simulink library "casper_library_downconverter"  (Simulink 7.0)
libraries: xbsIndex_r4 x81, casper_library_downconverter x18, casper_library_misc x1
(part 1 of 2)
settings Model: Creator=mdexter  LastModifiedBy=mdexter

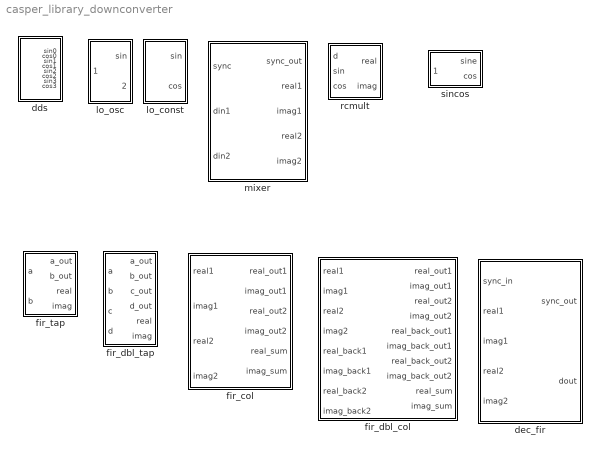
== system casper_library_downconverter ==
  dds : Subsystem  mask(dds){freq_div=4, freq=1, num_lo=4, n_bits=8, latency=2}
      mask prompts: freq_div "Frequency divisions (M)"; freq "Frequency (? / M*2pi)"; num_lo "Parallel LOs"; n_bits "Bit Width"
      mask help:
      | Generates P channels of sin and cos data for mixing
      | with input data in a DDC. To generate frequency
      | N/M(Fc x P) (where Fc is the clock rate)
      | M = "Frequency Divisions", N = "Frequency",
      | Parallel LOs = P
      mask init:
      | dds_init(gcb, ...
      |     'freq_div', freq_div, ...
      |     'freq', freq, ...
      |     'num_lo', num_lo, ...
      |     'n_bits', n_bits, ...
      |     'latency', latency);
      settings: AttributesFormatString=lo at -1/4
      mask Help: eval('xlWeb(''http://casper.berkeley.edu/wiki/Dds'')')
  dec_fir : Subsystem  mask(dec_fir){n_inputs=2, coeff=getfield( getfield( get_param( gcb,'UserData' ), 'parameters'),'coeff'), n_bits=4, quantization=Truncate, add_latency=1, mult_latency=2, coeff_bit_width=25, coeff_bin_pt=24, adder_tree_hdl=on}
      mask prompts: n_inputs "Number of Parallel Streams"; coeff "Coefficients"; n_bits "Bit Width Out"; quantization "Quantization Behavior"; add_latency "Add Latency"; mult_latency "Mult Latency"; coeff_bit_width "Coefficient bit width"; coeff_bin_pt "Coefficient binary point"; adder_tree_hdl "Implement first stage of adder trees after multiplication as behavioural HDL"
      mask help: FIR filter which can handle multiple time samples in parallel and decimates down to 1 time sample. If coefficients are symmetric, will automatically fold before multiplying.
      mask init:
      | dec_fir_init(gcb, ...
      |     'n_inputs', n_inputs, ...
      |     'coeff', coeff, ...
      |     'n_bits', n_bits, ...
      |     'quantization', quantization, ...
      |     'add_latency', add_latency, ...
      |     'mult_latency', mult_latency, ...
      |     'coeff_bit_width', coeff_bit_width, ...
      |     'coeff_bin_pt', coeff_bin_pt, ...
      |     'adder_tree_hdl', adder_tree_hdl);
      settings: AttributesFormatString=|
      | 8 taps
      | 4_3 r/i
      mask Help: eval('xlWeb(''http://casper.berkeley.edu/wiki/Dec_fir'')')
      mask StyleString: edit,edit,edit,popup(Truncate|Round  (unbiased: +/- Inf)|Round  (unbiased: Even Values)),edit,edit,edit,edit,checkbox
  fir_col : Subsystem  mask(fir_col){n_inputs=2, coeff=[2 3], add_latency=1, mult_latency=2, coeff_bit_width=25, coeff_bin_pt=24, adder_tree_hdl=off}
      mask prompts: n_inputs "Inputs"; coeff "Coefficients"; add_latency "Add latency"; mult_latency "Mult Latency"; coeff_bit_width "Coefficient bit width"; coeff_bin_pt "Coefficient binary point"; adder_tree_hdl "Implement first stage of adder trees on output as behavioural HDL"
      mask init:
      | fir_col_init(gcb, ...
      |     'n_inputs', n_inputs,...
      |     'coeff', coeff, ...
      |     'mult_latency', mult_latency, ...
      |     'add_latency', add_latency, ...
      |     'coeff_bit_width', coeff_bit_width, ...
      |     'coeff_bin_pt', coeff_bin_pt, ...
      |     'adder_tree_hdl', adder_tree_hdl);
      mask Help: eval('xlWeb(''http://casper.berkeley.edu/wiki/Fir_col'')')
  fir_dbl_col : Subsystem  mask(fir_dbl_col){n_inputs=2, coeff=[0.1 0.2 0.3 0.4], add_latency=1, mult_latency=2, coeff_bit_width=25, coeff_bin_pt=24, adder_tree_hdl=off}
      mask prompts: n_inputs "Inputs"; coeff "Coefficients"; add_latency "Add latency"; mult_latency "Mult Latency"; coeff_bit_width "Coefficient bit width"; coeff_bin_pt "Coefficient binary point"; adder_tree_hdl "Implement first stage of adder trees on output as behavioural HDL"
      mask init:
      | fir_dbl_col_init(gcb, ...
      |     'n_inputs', n_inputs, ...
      |     'coeff', coeff, ...
      |     'mult_latency', mult_latency, ...
      |     'add_latency', add_latency, ...
      |     'coeff_bit_width', coeff_bit_width, ...
      |     'coeff_bin_pt', coeff_bin_pt,  ...
      |     'adder_tree_hdl', adder_tree_hdl);
      mask Help: eval('xlWeb(''http://casper.berkeley.edu/wiki/Fir_dbl_col'')')
  fir_dbl_tap : Subsystem  mask(fir_dbl_tap){factor=0.073384, add_latency=1, mult_latency=2, coeff_bit_width=18, coeff_bin_pt=17}
      mask prompts: add_latency "Add latency"; mult_latency "Mult latency"; coeff_bit_width "Coefficient bit width"; coeff_bin_pt "Coefficient binary point"
      mask Help: eval('xlWeb(''http://casper.berkeley.edu/wiki/Fir_dbl_tap'')')
  fir_tap : Subsystem  mask(fir_tap){factor=1, latency=2, coeff_bit_width=25, coeff_bin_pt=24}
      mask prompts: latency "Mult latency"; coeff_bit_width "Coefficient bit width"; coeff_bin_pt "Coefficient binary point"
      mask help: Multiplies input data with factor specified.
      mask Help: eval('xlWeb(''http://casper.berkeley.edu/wiki/Fir_tap'')')
  lo_const : Subsystem  mask(lo_const){n_bits=18, phase=0}
      mask prompts: n_bits "Output Bitwidth"; phase "Phase (0 to 2*pi)"
      mask help:
      | Generates a complex constant associated with the
      | phase supplied as a parameter.
      mask Help: eval('xlWeb(''http://casper.berkeley.edu/wiki/Lo_const'')')
  lo_osc : Subsystem  mask(lo_osc){n_bits=7, counter_step=3, counter_start=4, counter_width=4, latency=2}
      mask prompts: n_bits "Output Bitwidth"; counter_step "counter step"; counter_start "counter start value"; counter_width "Counter Bitwidth"; latency "Lookup latency"
      mask help:
      | Generates -sin and cos data using a look-up
      | table.
      mask init:
      | lo_osc_init(gcb, ...
      |     'n_bits', n_bits, ...
      |     'counter_step', counter_step, ...
      |     'counter_start', counter_start, ...
      |     'counter_width', counter_width, ...
      |     'latency', latency);
      mask Help: eval('xlWeb(''http://casper.berkeley.edu/wiki/Lo_osc'')')
  mixer : Subsystem  mask(mixer){freq_div=2, freq=2, nstreams=2, n_bits=4, bram_latency=2, mult_latency=4}
      mask prompts: freq_div "Frequency Divisions (M)"; freq "Mixing Frequency (? / M*2pi)"; nstreams "Number of Parallel Streams"; n_bits "Bit Width"; bram_latency "BRAM Latency"; mult_latency "Mult Latency"
      mask help: Digitally mixes an input signal (which can be several samples in parallel) with an LO of the indicated frequency (which is some fraction of the native FPGA clock rate).
      mask init:
      | mixer_init(gcb, ...
      |     'freq_div', freq_div, ...
      |     'freq', freq, ...
      |     'nstreams', nstreams, ...
      |     'n_bits', n_bits, ...
      |     'bram_latency', bram_latency, ...
      |     'mult_latency', mult_latency);
      settings: AttributesFormatString=lo at -2/2
      mask Help: eval('xlWeb(''http://casper.berkeley.edu/wiki/Mixer'')')
  rcmult : Subsystem  mask(rcmult){latency=3}
      mask prompts: latency "Multiplier latency"
      mask help:
      | Multiplies input data with cos and sin inputs and
      | outputs results on real and imag ports
      | respectively.
      mask Help: eval('xlWeb(''http://casper.berkeley.edu/wiki/Rcmult'')')
  sincos : Subsystem  mask(sincos){func=sine and cosine, neg_sin=off, neg_cos=off, symmetric=on, handle_sync=off, depth_bits=10, bit_width=16, bram_latency=2}
      mask prompts: func "Function"; neg_sin "Negative sine"; neg_cos "Negative cosine"; symmetric "Symmetric output"; handle_sync "Handle sync"; depth_bits "Lookup table depth (2^?)"; bit_width "Output bit width"; bram_latency "BRAM latency"
      mask init:
      | sincos_init(gcb, ...
      |     'func', func, ...
      |     'neg_sin', neg_sin, ...
      |     'neg_cos', neg_cos, ...
      |     'symmetric', symmetric, ...
      |     'handle_sync', handle_sync, ...
      |     'depth_bits', depth_bits, ...
      |     'bit_width', bit_width, ...
      |     'bram_latency', bram_latency);
      mask StyleString: popup(cosine|sine|sine and cosine),checkbox,checkbox,checkbox,checkbox,edit,edit,edit

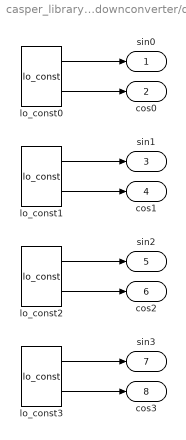
== system casper_library_downconverter/dds ==
  lo_const0 : casper_library_downconverter/lo_const  SystemSampleTime=-1  n_bits=8  phase=0
  lo_const1 : casper_library_downconverter/lo_const  SystemSampleTime=-1  n_bits=8  phase=1.5708
  lo_const2 : casper_library_downconverter/lo_const  SystemSampleTime=-1  n_bits=8  phase=3.1416
  lo_const3 : casper_library_downconverter/lo_const  SystemSampleTime=-1  n_bits=8  phase=4.7124
  sin0 : Outport  OutDataType=sfix(16)  OutScaling=2^0
  cos0 : Outport  Port=2  OutDataType=sfix(16)  OutScaling=2^0
  sin1 : Outport  Port=3  OutDataType=sfix(16)  OutScaling=2^0
  cos1 : Outport  Port=4  OutDataType=sfix(16)  OutScaling=2^0
  sin2 : Outport  Port=5  OutDataType=sfix(16)  OutScaling=2^0
  cos2 : Outport  Port=6  OutDataType=sfix(16)  OutScaling=2^0
  sin3 : Outport  Port=7  OutDataType=sfix(16)  OutScaling=2^0
  cos3 : Outport  Port=8  OutDataType=sfix(16)  OutScaling=2^0
  wires:
  lo_const3/2 -> cos3/1
  lo_const3/1 -> sin3/1
  lo_const2/2 -> cos2/1
  lo_const2/1 -> sin2/1
  lo_const1/2 -> cos1/1
  lo_const1/1 -> sin1/1
  lo_const0/2 -> cos0/1
  lo_const0/1 -> sin0/1

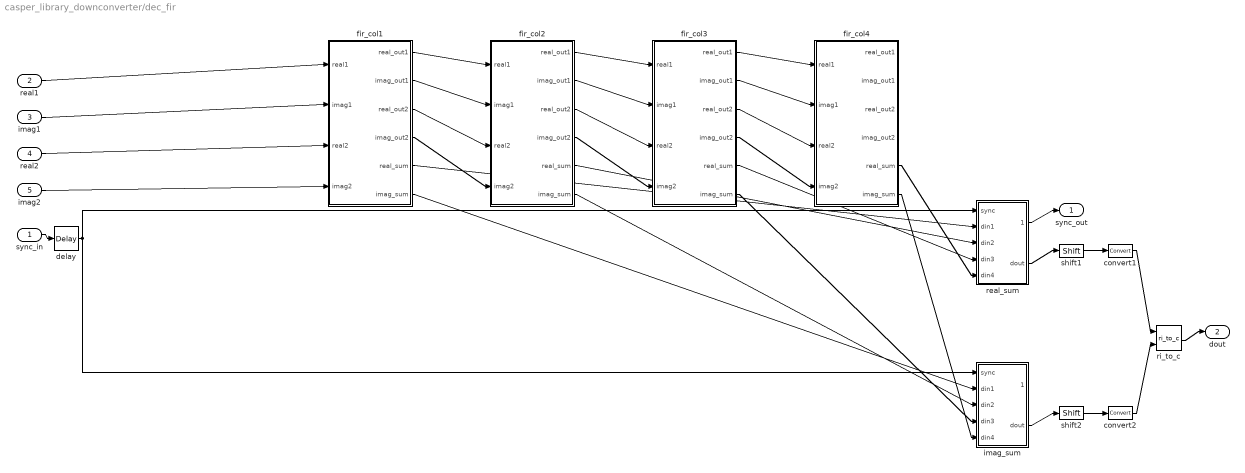
== system casper_library_downconverter/dec_fir ==
  sync_in : Inport
  real1 : Inport  Port=2
  imag1 : Inport  Port=3
  real2 : Inport  Port=4
  imag2 : Inport  Port=5
  convert1 : xbsIndex_r4/Convert  arith_type="Signed  (2's comp)"  n_bits=4  bin_pt=3  quantization=Truncate  overflow=Wrap  latency=1  dbl_ovrd=off  pipeline=off  block_type=convert
      settings: block_version=10.1.3
  convert2 : xbsIndex_r4/Convert  arith_type="Signed  (2's comp)"  n_bits=4  bin_pt=3  quantization=Truncate  overflow=Wrap  latency=1  dbl_ovrd=off  pipeline=off  block_type=convert
      settings: block_version=10.1.3
  delay : xbsIndex_r4/Delay  en=off  latency=4  dbl_ovrd=off  reg_retiming=off  block_type=delay
  fir_col1 : Subsystem  AncestorBlock=casper_library_downconverter/fir_col  mask(fir_col){n_inputs=2, coeff=[0.20000000000000001110223024625157     0.10000000000000000555111512312578], add_latency=1, mult_latency=2, coeff_bit_width=25, coeff_bin_pt=24, adder_tree_hdl=on}
      mask prompts: n_inputs "Inputs"; coeff "Coefficients"; add_latency "Add latency"; mult_latency "Mult Latency"; coeff_bit_width "Coefficient bit width"; coeff_bin_pt "Coefficient binary point"; adder_tree_hdl "Implement first stage of adder trees on output as behavioural HDL"
      mask init: same as casper_library_downconverter/fir_col
      mask Help: eval('xlWeb(''http://casper.berkeley.edu/wiki/Fir_col'')')
  fir_col2 : Subsystem  AncestorBlock=casper_library_downconverter/fir_col  mask(fir_col){n_inputs=2, coeff=[0.40000000000000002220446049250313     0.29999999999999998889776975374843], add_latency=1, mult_latency=2, coeff_bit_width=25, coeff_bin_pt=24, adder_tree_hdl=on}
      mask prompts: n_inputs "Inputs"; coeff "Coefficients"; add_latency "Add latency"; mult_latency "Mult Latency"; coeff_bit_width "Coefficient bit width"; coeff_bin_pt "Coefficient binary point"; adder_tree_hdl "Implement first stage of adder trees on output as behavioural HDL"
      mask init: same as casper_library_downconverter/fir_col
      mask Help: eval('xlWeb(''http://casper.berkeley.edu/wiki/Fir_col'')')
  fir_col3 : Subsystem  AncestorBlock=casper_library_downconverter/fir_col  mask(fir_col){n_inputs=2, coeff=[0.59999999999999997779553950749687                                    0.5], add_latency=1, mult_latency=2, coeff_bit_width=25, coeff_bin_pt=24, adder_tree_hdl=on}
      mask prompts: n_inputs "Inputs"; coeff "Coefficients"; add_latency "Add latency"; mult_latency "Mult Latency"; coeff_bit_width "Coefficient bit width"; coeff_bin_pt "Coefficient binary point"; adder_tree_hdl "Implement first stage of adder trees on output as behavioural HDL"
      mask init: same as casper_library_downconverter/fir_col
      mask Help: eval('xlWeb(''http://casper.berkeley.edu/wiki/Fir_col'')')
  fir_col4 : Subsystem  AncestorBlock=casper_library_downconverter/fir_col  mask(fir_col){n_inputs=2, coeff=[0.80000000000000004440892098500626     0.69999999999999995559107901499374], add_latency=1, mult_latency=2, coeff_bit_width=25, coeff_bin_pt=24, adder_tree_hdl=on}
      mask prompts: n_inputs "Inputs"; coeff "Coefficients"; add_latency "Add latency"; mult_latency "Mult Latency"; coeff_bit_width "Coefficient bit width"; coeff_bin_pt "Coefficient binary point"; adder_tree_hdl "Implement first stage of adder trees on output as behavioural HDL"
      mask init: same as casper_library_downconverter/fir_col
      mask Help: eval('xlWeb(''http://casper.berkeley.edu/wiki/Fir_col'')')
  imag_sum : Subsystem  AncestorBlock=casper_library_misc/adder_tree  mask(adder_tree){n_inputs=4, latency=1, first_stage_hdl=off, behavioral=off}
      mask prompts: n_inputs "Number of Inputs"; latency "Add Latency"; first_stage_hdl "Use behavioural HDL for first stage of adders"; behavioral "Use behavioral HDL for all adders"
      mask help:
      | Sums all inputs using a tree of adds and delays.
      |
      | Number of inputs: The number of inputs to the block to be summed
      | Add latency: The number of clock cycles to perform one addition (affects timing).
      | Use behavioural HDL for first stage of adders: Causes the first stage of adders to be absorbed into DSP blocks if multipliers precede them (Virtex 5).
      | Use behavioural HDL for all adders: Causes all adders in all stages to be implemented in behavioural HDL (may improve timing).
      mask init:
      | adder_tree_init(gcb, ...
      |     'n_inputs', n_inputs, ...
      |     'latency', latency, ...
      |     'first_stage_hdl', first_stage_hdl, ...
      |     'behavioral', behavioral);
      settings: AttributesFormatString=latency 2
      mask Help: eval('xlWeb(''http://casper.berkeley.edu/wiki/Adder_tree'')')
  real_sum : Subsystem  AncestorBlock=casper_library_misc/adder_tree  mask(adder_tree){n_inputs=4, latency=1, first_stage_hdl=off, behavioral=off}
      mask prompts: n_inputs "Number of Inputs"; latency "Add Latency"; first_stage_hdl "Use behavioural HDL for first stage of adders"; behavioral "Use behavioral HDL for all adders"
      mask help:
      | Sums all inputs using a tree of adds and delays.
      |
      | Number of inputs: The number of inputs to the block to be summed
      | Add latency: The number of clock cycles to perform one addition (affects timing).
      | Use behavioural HDL for first stage of adders: Causes the first stage of adders to be absorbed into DSP blocks if multipliers precede them (Virtex 5).
      | Use behavioural HDL for all adders: Causes all adders in all stages to be implemented in behavioural HDL (may improve timing).
      mask init:
      | adder_tree_init(gcb, ...
      |     'n_inputs', n_inputs, ...
      |     'latency', latency, ...
      |     'first_stage_hdl', first_stage_hdl, ...
      |     'behavioral', behavioral);
      settings: AttributesFormatString=latency 2
      mask Help: eval('xlWeb(''http://casper.berkeley.edu/wiki/Adder_tree'')')
  ri_to_c : casper_library_misc/ri_to_c  SystemSampleTime=-1
  shift1 : xbsIndex_r4/Shift  shift_dir=Left  shift_bits=1  en=off  latency=0  precision=Full  arith_type="Signed  (2's comp)"  n_bits=16  bin_pt=14  quantization=Truncate  overflow=Wrap  dbl_ovrd=off  block_type=shift
      settings: block_version=10.1.3
  shift2 : xbsIndex_r4/Shift  shift_dir=Left  shift_bits=1  en=off  latency=0  precision=Full  arith_type="Signed  (2's comp)"  n_bits=16  bin_pt=14  quantization=Truncate  overflow=Wrap  dbl_ovrd=off  block_type=shift
      settings: block_version=10.1.3
  sync_out : Outport
  dout : Outport  Port=2
  wires:
  real_sum/1(sync_out) -> sync_out/1
  delay/1 -> imag_sum/1(sync), real_sum/1(sync)
  sync_in/1 -> delay/1
  ri_to_c/1 -> dout/1
  convert2/1 -> ri_to_c/2
  convert1/1 -> ri_to_c/1
  shift2/1 -> convert2/1
  shift1/1 -> convert1/1
  imag_sum/2(dout) -> shift2/1
  real_sum/2(dout) -> shift1/1
  fir_col4/6(imag_sum) -> imag_sum/5(din4)
  fir_col4/5(real_sum) -> real_sum/5(din4)
  fir_col3/4(imag_out2) -> fir_col4/4(imag2)
  fir_col3/3(real_out2) -> fir_col4/3(real2)
  fir_col3/2(imag_out1) -> fir_col4/2(imag1)
  fir_col3/1(real_out1) -> fir_col4/1(real1)
  fir_col3/6(imag_sum) -> imag_sum/4(din3)
  fir_col3/5(real_sum) -> real_sum/4(din3)
  fir_col2/4(imag_out2) -> fir_col3/4(imag2)
  fir_col2/3(real_out2) -> fir_col3/3(real2)
  fir_col2/2(imag_out1) -> fir_col3/2(imag1)
  fir_col2/1(real_out1) -> fir_col3/1(real1)
  fir_col2/6(imag_sum) -> imag_sum/3(din2)
  fir_col2/5(real_sum) -> real_sum/3(din2)
  fir_col1/4(imag_out2) -> fir_col2/4(imag2)
  fir_col1/3(real_out2) -> fir_col2/3(real2)
  fir_col1/2(imag_out1) -> fir_col2/2(imag1)
  fir_col1/1(real_out1) -> fir_col2/1(real1)
  fir_col1/6(imag_sum) -> imag_sum/2(din1)
  fir_col1/5(real_sum) -> real_sum/2(din1)
  imag2/1 -> fir_col1/4(imag2)
  real2/1 -> fir_col1/3(real2)
  imag1/1 -> fir_col1/2(imag1)
  real1/1 -> fir_col1/1(real1)

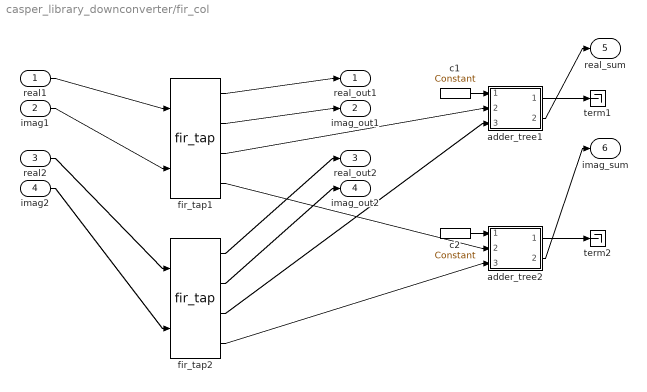
== system casper_library_downconverter/fir_col ==
  real1 : Inport
  imag1 : Inport  Port=2
  real2 : Inport  Port=3
  imag2 : Inport  Port=4
  adder_tree1 : Subsystem  AncestorBlock=casper_library_misc/adder_tree  mask(adder_tree){n_inputs=2, latency=1, first_stage_hdl=off, behavioral=off}
      mask prompts: n_inputs "Number of Inputs"; latency "Add Latency"; first_stage_hdl "Use behavioural HDL for first stage of adders"; behavioral "Use behavioral HDL for all adders"
      mask help:
      | Sums all inputs using a tree of adds and delays.
      |
      | Number of inputs: The number of inputs to the block to be summed
      | Add latency: The number of clock cycles to perform one addition (affects timing).
      | Use behavioural HDL for first stage of adders: Causes the first stage of adders to be absorbed into DSP blocks if multipliers precede them (Virtex 5).
      | Use behavioural HDL for all adders: Causes all adders in all stages to be implemented in behavioural HDL (may improve timing).
      mask init:
      | adder_tree_init(gcb, ...
      |     'n_inputs', n_inputs, ...
      |     'latency', latency, ...
      |     'first_stage_hdl', first_stage_hdl, ...
      |     'behavioral', behavioral);
      settings: AttributesFormatString=latency 1
      mask Help: eval('xlWeb(''http://casper.berkeley.edu/wiki/Adder_tree'')')
  adder_tree2 : Subsystem  AncestorBlock=casper_library_misc/adder_tree  mask(adder_tree){n_inputs=2, latency=1, first_stage_hdl=off, behavioral=off}
      mask prompts: n_inputs "Number of Inputs"; latency "Add Latency"; first_stage_hdl "Use behavioural HDL for first stage of adders"; behavioral "Use behavioral HDL for all adders"
      mask help:
      | Sums all inputs using a tree of adds and delays.
      |
      | Number of inputs: The number of inputs to the block to be summed
      | Add latency: The number of clock cycles to perform one addition (affects timing).
      | Use behavioural HDL for first stage of adders: Causes the first stage of adders to be absorbed into DSP blocks if multipliers precede them (Virtex 5).
      | Use behavioural HDL for all adders: Causes all adders in all stages to be implemented in behavioural HDL (may improve timing).
      mask init:
      | adder_tree_init(gcb, ...
      |     'n_inputs', n_inputs, ...
      |     'latency', latency, ...
      |     'first_stage_hdl', first_stage_hdl, ...
      |     'behavioral', behavioral);
      settings: AttributesFormatString=latency 1
      mask Help: eval('xlWeb(''http://casper.berkeley.edu/wiki/Adder_tree'')')
  c1 : xbsIndex_r4/Constant  arith_type=Signed (2's comp)  const=1  n_bits=16  bin_pt=14  explicit_period=on  period=1  equ=P=C  opselect=C  inp2=PCIN>>17  opr=+  inp1=P  carry=CIN  dbl_ovrd=off  block_type=constant
  c2 : xbsIndex_r4/Constant  arith_type=Signed (2's comp)  const=1  n_bits=16  bin_pt=14  explicit_period=on  period=1  equ=P=C  opselect=C  inp2=PCIN>>17  opr=+  inp1=P  carry=CIN  dbl_ovrd=off  block_type=constant
  fir_tap1 : casper_library_downconverter/fir_tap  SystemSampleTime=-1  factor=2  latency=2  coeff_bit_width=25  coeff_bin_pt=24
  fir_tap2 : casper_library_downconverter/fir_tap  SystemSampleTime=-1  factor=3  latency=2  coeff_bit_width=25  coeff_bin_pt=24
  term1 : Terminator
  term2 : Terminator
  real_out1 : Outport
  imag_out1 : Outport  Port=2
  real_out2 : Outport  Port=3
  imag_out2 : Outport  Port=4
  real_sum : Outport  Port=5
  imag_sum : Outport  Port=6
  wires:
  adder_tree1/1(sync_out) -> term1/1
  adder_tree2/1(sync_out) -> term2/1
  c1/1 -> adder_tree1/1(sync)
  c2/1 -> adder_tree2/1(sync)
  adder_tree1/2(dout) -> real_sum/1
  adder_tree2/2(dout) -> imag_sum/1
  real1/1 -> fir_tap1/1
  imag1/1 -> fir_tap1/2
  fir_tap1/1 -> real_out1/1
  fir_tap1/2 -> imag_out1/1
  fir_tap1/3 -> adder_tree1/2(din1)
  fir_tap1/4 -> adder_tree2/2(din1)
  real2/1 -> fir_tap2/1
  imag2/1 -> fir_tap2/2
  fir_tap2/1 -> real_out2/1
  fir_tap2/2 -> imag_out2/1
  fir_tap2/3 -> adder_tree1/3(din2)
  fir_tap2/4 -> adder_tree2/3(din2)

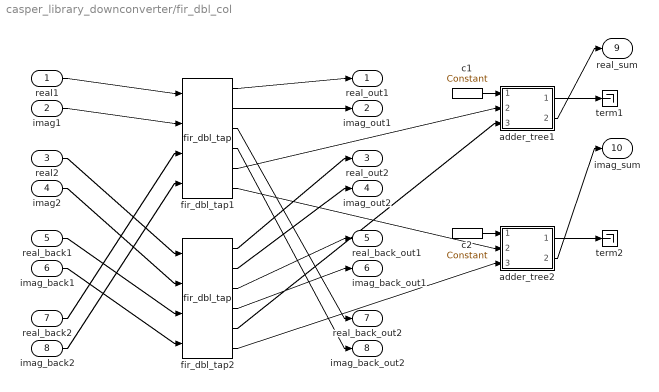
== system casper_library_downconverter/fir_dbl_col ==
  real1 : Inport
  imag1 : Inport  Port=2
  real2 : Inport  Port=3
  imag2 : Inport  Port=4
  real_back1 : Inport  Port=5
  imag_back1 : Inport  Port=6
  real_back2 : Inport  Port=7
  imag_back2 : Inport  Port=8
  adder_tree1 : Subsystem  AncestorBlock=casper_library_misc/adder_tree  mask(adder_tree){n_inputs=2, latency=1, first_stage_hdl=off, behavioral=off}
      mask prompts: n_inputs "Number of Inputs"; latency "Add Latency"; first_stage_hdl "Use behavioural HDL for first stage of adders"; behavioral "Use behavioral HDL for all adders"
      mask help:
      | Sums all inputs using a tree of adds and delays.
      |
      | Number of inputs: The number of inputs to the block to be summed
      | Add latency: The number of clock cycles to perform one addition (affects timing).
      | Use behavioural HDL for first stage of adders: Causes the first stage of adders to be absorbed into DSP blocks if multipliers precede them (Virtex 5).
      | Use behavioural HDL for all adders: Causes all adders in all stages to be implemented in behavioural HDL (may improve timing).
      mask init:
      | adder_tree_init(gcb, ...
      |     'n_inputs', n_inputs, ...
      |     'latency', latency, ...
      |     'first_stage_hdl', first_stage_hdl, ...
      |     'behavioral', behavioral);
      settings: AttributesFormatString=latency 1
      mask Help: eval('xlWeb(''http://casper.berkeley.edu/wiki/Adder_tree'')')
  adder_tree2 : Subsystem  AncestorBlock=casper_library_misc/adder_tree  mask(adder_tree){n_inputs=2, latency=1, first_stage_hdl=off, behavioral=off}
      mask prompts: n_inputs "Number of Inputs"; latency "Add Latency"; first_stage_hdl "Use behavioural HDL for first stage of adders"; behavioral "Use behavioral HDL for all adders"
      mask help:
      | Sums all inputs using a tree of adds and delays.
      |
      | Number of inputs: The number of inputs to the block to be summed
      | Add latency: The number of clock cycles to perform one addition (affects timing).
      | Use behavioural HDL for first stage of adders: Causes the first stage of adders to be absorbed into DSP blocks if multipliers precede them (Virtex 5).
      | Use behavioural HDL for all adders: Causes all adders in all stages to be implemented in behavioural HDL (may improve timing).
      mask init:
      | adder_tree_init(gcb, ...
      |     'n_inputs', n_inputs, ...
      |     'latency', latency, ...
      |     'first_stage_hdl', first_stage_hdl, ...
      |     'behavioral', behavioral);
      settings: AttributesFormatString=latency 1
      mask Help: eval('xlWeb(''http://casper.berkeley.edu/wiki/Adder_tree'')')
  c1 : xbsIndex_r4/Constant  arith_type=Signed (2's comp)  const=1  n_bits=16  bin_pt=14  explicit_period=on  period=1  equ=P=C  opselect=C  inp2=PCIN>>17  opr=+  inp1=P  carry=CIN  dbl_ovrd=off  block_type=constant
  c2 : xbsIndex_r4/Constant  arith_type=Signed (2's comp)  const=1  n_bits=16  bin_pt=14  explicit_period=on  period=1  equ=P=C  opselect=C  inp2=PCIN>>17  opr=+  inp1=P  carry=CIN  dbl_ovrd=off  block_type=constant
  fir_dbl_tap1 : casper_library_downconverter/fir_dbl_tap  SystemSampleTime=-1  factor=0.1  add_latency=1  mult_latency=2  coeff_bit_width=25  coeff_bin_pt=24
  fir_dbl_tap2 : casper_library_downconverter/fir_dbl_tap  SystemSampleTime=-1  factor=0.2  add_latency=1  mult_latency=2  coeff_bit_width=25  coeff_bin_pt=24
  term1 : Terminator
  term2 : Terminator
  real_out1 : Outport
  imag_out1 : Outport  Port=2
  real_out2 : Outport  Port=3
  imag_out2 : Outport  Port=4
  real_back_out1 : Outport  Port=5
  imag_back_out1 : Outport  Port=6
  real_back_out2 : Outport  Port=7
  imag_back_out2 : Outport  Port=8
  real_sum : Outport  Port=9
  imag_sum : Outport  Port=10
  wires:
  adder_tree1/1(sync_out) -> term1/1
  adder_tree2/1(sync_out) -> term2/1
  c1/1 -> adder_tree1/1(sync)
  c2/1 -> adder_tree2/1(sync)
  adder_tree1/2(dout) -> real_sum/1
  adder_tree2/2(dout) -> imag_sum/1
  real1/1 -> fir_dbl_tap1/1
  imag1/1 -> fir_dbl_tap1/2
  real_back2/1 -> fir_dbl_tap1/3
  imag_back2/1 -> fir_dbl_tap1/4
  fir_dbl_tap1/1 -> real_out1/1
  fir_dbl_tap1/2 -> imag_out1/1
  fir_dbl_tap1/3 -> real_back_out2/1
  fir_dbl_tap1/4 -> imag_back_out2/1
  fir_dbl_tap1/5 -> adder_tree1/2(din1)
  fir_dbl_tap1/6 -> adder_tree2/2(din1)
  real2/1 -> fir_dbl_tap2/1
  imag2/1 -> fir_dbl_tap2/2
  real_back1/1 -> fir_dbl_tap2/3
  imag_back1/1 -> fir_dbl_tap2/4
  fir_dbl_tap2/1 -> real_out2/1
  fir_dbl_tap2/2 -> imag_out2/1
  fir_dbl_tap2/3 -> real_back_out1/1
  fir_dbl_tap2/4 -> imag_back_out1/1
  fir_dbl_tap2/5 -> adder_tree1/3(din2)
  fir_dbl_tap2/6 -> adder_tree2/3(din2)

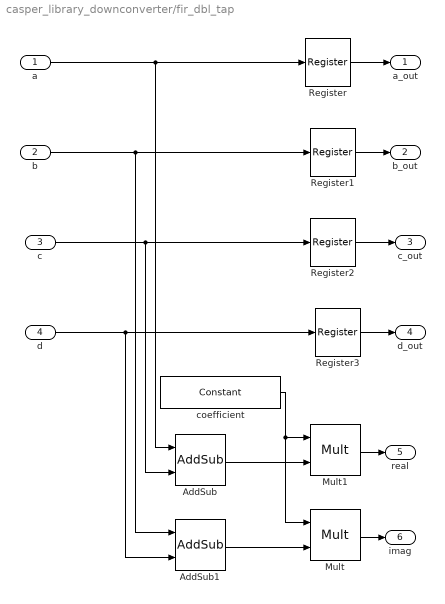
== system casper_library_downconverter/fir_dbl_tap ==
  a : Inport  OutDataType=sfix(16)  OutScaling=2^0
  b : Inport  Port=2  OutDataType=sfix(16)  OutScaling=2^0
  c : Inport  Port=3  OutDataType=sfix(16)  OutScaling=2^0
  d : Inport  Port=4  OutDataType=sfix(16)  OutScaling=2^0
  AddSub : xbsIndex_r4/AddSub  mode=Addition  use_carryin=off  use_carryout=off  en=off  latency=add_latency  precision=Full  arith_type="Signed  (2's comp)"  n_bits=18  bin_pt=16  quantization=Truncate  overflow=Wrap  dbl_ovrd=off  use_behavioral_HDL=on  pipelined=off  use_rpm=on  hw_selection=Fabric  block_type=addsub
      settings: xl_area=[0, 0, 0, 0, 0, 0, 0]  block_version=9.2.01
  AddSub1 : xbsIndex_r4/AddSub  mode=Addition  use_carryin=off  use_carryout=off  en=off  latency=add_latency  precision=Full  arith_type="Signed  (2's comp)"  n_bits=18  bin_pt=16  quantization=Truncate  overflow=Wrap  dbl_ovrd=off  use_behavioral_HDL=on  pipelined=off  use_rpm=on  hw_selection=Fabric  block_type=addsub
      settings: xl_area=[0, 0, 0, 0, 0, 0, 0]  block_version=9.2.01
  Mult : xbsIndex_r4/Mult  precision=Full  arith_type="Signed  (2's comp)"  n_bits=18  bin_pt=17  quantization=Truncate  overflow=Wrap  en=off  latency=mult_latency  dbl_ovrd=off  use_behavioral_HDL=on  use_embedded=on  opt=Speed  optimum_pipeline=off  pipeline=on  use_rpm=off  placement_style=Rectangular shape  block_type=mult
      settings: infoedit=Hardware notes: To use the internal pipeline stage of the dedicated multiplier you must select 'Pipeline for maximum performance'.  xl_area=[0, 0, 0, 0, 0, 0, 0]  block_version=9.2.01
  Mult1 : xbsIndex_r4/Mult  precision=Full  arith_type="Signed  (2's comp)"  n_bits=18  bin_pt=17  quantization=Truncate  overflow=Wrap  en=off  latency=mult_latency  dbl_ovrd=off  use_behavioral_HDL=on  use_embedded=on  opt=Speed  optimum_pipeline=off  pipeline=on  use_rpm=off  placement_style=Rectangular shape  block_type=mult
      settings: infoedit=Hardware notes: To use the internal pipeline stage of the dedicated multiplier you must select 'Pipeline for maximum performance'.  xl_area=[0, 0, 0, 0, 0, 0, 0]  block_version=9.2.01
  Register{,1..3} (4 alike) : xbsIndex_r4/Register  init=0  rst=off  en=off  dbl_ovrd=off  block_type=register
      settings: xl_area=[0, 0, 0, 0, 0, 0, 0]  block_version=9.2.01
  coefficient : xbsIndex_r4/Constant  arith_type=Signed (2's comp)  const=factor  n_bits=coeff_bit_width  bin_pt=coeff_bin_pt  explicit_period=on  period=1  equ=P=C  opselect=C  inp2=PCIN>>17  opr=+  inp1=P  carry=CIN  dbl_ovrd=off  block_type=constant
      settings: block_version=9.2.01
  a_out : Outport  OutDataType=sfix(16)  OutScaling=2^0
  b_out : Outport  Port=2  OutDataType=sfix(16)  OutScaling=2^0
  c_out : Outport  Port=3  OutDataType=sfix(16)  OutScaling=2^0
  d_out : Outport  Port=4  OutDataType=sfix(16)  OutScaling=2^0
  real : Outport  Port=5  OutDataType=sfix(16)  OutScaling=2^0
  imag : Outport  Port=6  OutDataType=sfix(16)  OutScaling=2^0
  wires:
  AddSub1/1 -> Mult/2
  AddSub/1 -> Mult1/2
  d/1 -> AddSub1/2, Register3/1
  c/1 -> AddSub/2, Register2/1
  b/1 -> AddSub1/1, Register1/1
  a/1 -> AddSub/1, Register/1
  Register2/1 -> c_out/1
  Register3/1 -> d_out/1
  Mult1/1 -> real/1
  Mult/1 -> imag/1
  coefficient/1 -> Mult1/1, Mult/1
  Register/1 -> a_out/1
  Register1/1 -> b_out/1

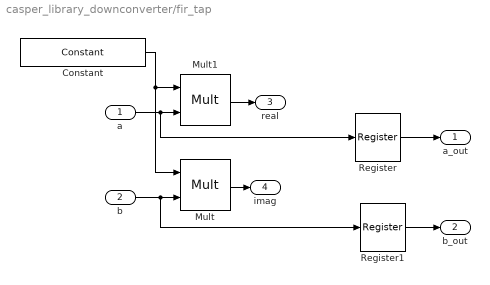
== system casper_library_downconverter/fir_tap ==
  a : Inport  OutDataType=sfix(16)  OutScaling=2^0
  b : Inport  Port=2  OutDataType=sfix(16)  OutScaling=2^0
  Constant : xbsIndex_r4/Constant  arith_type=Signed (2's comp)  const=factor  n_bits=coeff_bit_width  bin_pt=coeff_bin_pt  explicit_period=on  period=1  equ=P=C  opselect=C  inp2=PCIN>>17  opr=+  inp1=P  carry=CIN  dbl_ovrd=off  block_type=constant
      settings: block_version=9.1.01
  Mult : xbsIndex_r4/Mult  precision=Full  arith_type="Signed  (2's comp)"  n_bits=18  bin_pt=17  quantization=Truncate  overflow=Wrap  en=off  latency=latency  dbl_ovrd=off  use_behavioral_HDL=on  use_embedded=on  opt=Speed  optimum_pipeline=off  pipeline=on  use_rpm=off  placement_style=Rectangular shape  block_type=mult
      settings: infoedit=Hardware notes: To use the internal pipeline stage of the dedicated multiplier you must select 'Pipeline for maximum performance'.  xl_area=[0, 0, 0, 0, 0, 0, 0]  block_version=9.1.01
  Mult1 : xbsIndex_r4/Mult  precision=Full  arith_type="Signed  (2's comp)"  n_bits=18  bin_pt=17  quantization=Truncate  overflow=Wrap  en=off  latency=latency  dbl_ovrd=off  use_behavioral_HDL=on  use_embedded=on  opt=Speed  optimum_pipeline=off  pipeline=on  use_rpm=off  placement_style=Rectangular shape  block_type=mult
      settings: infoedit=Hardware notes: To use the internal pipeline stage of the dedicated multiplier you must select 'Pipeline for maximum performance'.  xl_area=[0, 0, 0, 0, 0, 0, 0]  block_version=9.1.01
  Register : xbsIndex_r4/Register  init=0  rst=off  en=off  dbl_ovrd=off  block_type=register
      settings: xl_area=[0, 0, 0, 0, 0, 0, 0]  block_version=9.1.01
  Register1 : xbsIndex_r4/Register  init=0  rst=off  en=off  dbl_ovrd=off  block_type=register
      settings: xl_area=[0, 0, 0, 0, 0, 0, 0]  block_version=9.1.01
  a_out : Outport  OutDataType=sfix(16)  OutScaling=2^0
  b_out : Outport  Port=2  OutDataType=sfix(16)  OutScaling=2^0
  real : Outport  Port=3  OutDataType=sfix(16)  OutScaling=2^0
  imag : Outport  Port=4  OutDataType=sfix(16)  OutScaling=2^0
  wires:
  Mult1/1 -> real/1
  b/1 -> Mult/2, Register1/1
  Mult/1 -> imag/1
  a/1 -> Mult1/2, Register/1
  Constant/1 -> Mult1/1, Mult/1
  Register/1 -> a_out/1
  Register1/1 -> b_out/1

== system casper_library_downconverter/lo_const ==
  const : xbsIndex_r4/Constant  arith_type=Signed (2's comp)  const=real(exp(phase*1j))  n_bits=n_bits  bin_pt=n_bits - 1  explicit_period=on  period=1  equ=P=C  opselect=C  inp2=PCIN>>17  opr=+  inp1=P  carry=CIN  dbl_ovrd=off  block_type=constant
      settings: block_version=9.1.01
  const1 : xbsIndex_r4/Constant  arith_type=Signed (2's comp)  const=-imag(exp(phase*1j))  n_bits=n_bits  bin_pt=n_bits - 1  explicit_period=on  period=1  equ=P=C  opselect=C  inp2=PCIN>>17  opr=+  inp1=P  carry=CIN  dbl_ovrd=off  block_type=constant
      settings: block_version=9.1.01
  sin : Outport  OutDataType=sfix(16)  OutScaling=2^0
  cos : Outport  Port=2  OutDataType=sfix(16)  OutScaling=2^0
  wires:
  const1/1 -> sin/1
  const/1 -> cos/1

== system casper_library_downconverter/lo_osc ==
  sync : Inport  OutDataType=sfix(16)  OutScaling=2^0
  counter : xbsIndex_r4/Counter  cnt_type=Free Running  cnt_to=Inf  operation=Up  start_count=counter_start  cnt_by_val=counter_step  arith_type=Unsigned  n_bits=counter_width  bin_pt=0  load_pin=off  rst=on  en=off  explicit_period=on  period=1  dbl_ovrd=off  use_behavioral_HDL=off  use_rpm=off  implementation=Fabric  block_type=counter
  sincos : Subsystem  AncestorBlock=casper_library_downconverter/sincos  mask(sincos){func=sine and cosine, neg_sin=on, neg_cos=off, symmetric=off, handle_sync=off, depth_bits=4, bit_width=7, bram_latency=2}
      mask prompts: func "Function"; neg_sin "Negative sine"; neg_cos "Negative cosine"; symmetric "Symmetric output"; handle_sync "Handle sync"; depth_bits "Lookup table depth (2^?)"; bit_width "Output bit width"; bram_latency "BRAM latency"
      mask init: same as casper_library_downconverter/sincos
      mask StyleString: popup(cosine|sine|sine and cosine),checkbox,checkbox,checkbox,checkbox,edit,edit,edit
  sin : Outport  OutDataType=sfix(16)  OutScaling=2^0
  cos : Outport  Port=2  OutDataType=sfix(16)  OutScaling=2^0
  wires:
  sync/1 -> counter/1
  counter/1 -> sincos/1(theta)
  sincos/2(cos) -> cos/1
  sincos/1(-sine) -> sin/1

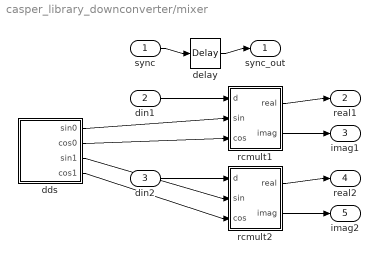
== system casper_library_downconverter/mixer ==
  sync : Inport  OutDataType=sfix(16)  OutScaling=2^0
  din1 : Inport  Port=2  OutDataType=sfix(16)  OutScaling=2^0
  din2 : Inport  Port=3  OutDataType=sfix(16)  OutScaling=2^0
  dds : Subsystem  AncestorBlock=casper_library_downconverter/dds  mask(dds){freq_div=2, freq=2, num_lo=2, n_bits=4, latency=2}
      mask prompts: freq_div "Frequency divisions (M)"; freq "Frequency (? / M*2pi)"; num_lo "Parallel LOs"; n_bits "Bit Width"
      mask init:
      | dds_init(gcb, ...
      |     'freq_div', freq_div, ...
      |     'freq', freq, ...
      |     'num_lo', num_lo, ...
      |     'n_bits', n_bits, ...
      |     'latency', latency);
      settings: AttributesFormatString=lo at -2/2
  delay : xbsIndex_r4/Delay  en=off  latency=4  dbl_ovrd=off  reg_retiming=off  block_type=delay
      settings: xl_area=[0, 0, 0, 0, 0, 0, 0]  block_version=9.1.01
  rcmult1 : Subsystem  AncestorBlock=casper_library_downconverter/rcmult  mask(rcmult){latency=4}
  rcmult2 : Subsystem  AncestorBlock=casper_library_downconverter/rcmult  mask(rcmult){latency=4}
  sync_out : Outport  OutDataType=sfix(16)  OutScaling=2^0
  real1 : Outport  Port=2  OutDataType=sfix(16)  OutScaling=2^0
  imag1 : Outport  Port=3  OutDataType=sfix(16)  OutScaling=2^0
  real2 : Outport  Port=4  OutDataType=sfix(16)  OutScaling=2^0
  imag2 : Outport  Port=5  OutDataType=sfix(16)  OutScaling=2^0
  wires:
  rcmult2/2(imag) -> imag2/1
  rcmult2/1(real) -> real2/1
  dds/4(cos1) -> rcmult2/3(cos)
  dds/3(sin1) -> rcmult2/2(sin)
  din2/1 -> rcmult2/1(d)
  rcmult1/2(imag) -> imag1/1
  rcmult1/1(real) -> real1/1
  dds/2(cos0) -> rcmult1/3(cos)
  dds/1(sin0) -> rcmult1/2(sin)
  din1/1 -> rcmult1/1(d)
  delay/1 -> sync_out/1
  sync/1 -> delay/1

== system casper_library_downconverter/rcmult ==
  d : Inport  OutDataType=sfix(16)  OutScaling=2^0
  sin : Inport  Port=2  OutDataType=sfix(16)  OutScaling=2^0
  cos : Inport  Port=3  OutDataType=sfix(16)  OutScaling=2^0
  Mult : xbsIndex_r4/Mult  precision=Full  arith_type="Signed  (2's comp)"  n_bits=8  bin_pt=2  quantization=Truncate  overflow=Wrap  en=off  latency=latency  dbl_ovrd=off  use_behavioral_HDL=off  use_embedded=on  opt=Speed  optimum_pipeline=off  pipeline=on  use_rpm=off  placement_style=Rectangular shape  block_type=mult
      settings: infoedit=Hardware notes: To use the internal pipeline stage of the dedicated multiplier you must select 'Pipeline for maximum performance'.  xl_area=[0, 0, 0, 0, 0, 0, 0]  block_version=9.1.01
  Mult1 : xbsIndex_r4/Mult  precision=Full  arith_type="Signed  (2's comp)"  n_bits=8  bin_pt=2  quantization=Truncate  overflow=Wrap  en=off  latency=latency  dbl_ovrd=off  use_behavioral_HDL=off  use_embedded=on  opt=Speed  optimum_pipeline=off  pipeline=on  use_rpm=off  placement_style=Rectangular shape  block_type=mult
      settings: infoedit=Hardware notes: To use the internal pipeline stage of the dedicated multiplier you must select 'Pipeline for maximum performance'.  xl_area=[0, 0, 0, 0, 0, 0, 0]  block_version=9.1.01
  real : Outport  OutDataType=sfix(16)  OutScaling=2^0
  imag : Outport  Port=2  OutDataType=sfix(16)  OutScaling=2^0
  wires:
  cos/1 -> Mult/2
  sin/1 -> Mult1/2
  d/1 -> Mult/1, Mult1/1
  Mult/1 -> real/1
  Mult1/1 -> imag/1

== system casper_library_downconverter/sincos ==
  theta : Inport
  rom0 : xbsIndex_r4/ROM  depth=2^depth_bits  initVector=sin(2*pi*(0:(2^depth_bits-1))/(2^depth_bits))  distributed_mem=Block RAM  rst=off  init_reg=0  en=off  latency=bram_latency  arith_type="Signed  (2's comp)"  n_bits=bit_width  bin_pt=bit_width-2  dbl_ovrd=off  optimize=Area  use_rpm=on  block_type=sprom
      settings: block_version=10.1.3
  rom1 : xbsIndex_r4/ROM  depth=2^depth_bits  initVector=cos(2*pi*(0:(2^depth_bits-1))/(2^depth_bits))  distributed_mem=Block RAM  rst=off  init_reg=0  en=off  latency=bram_latency  arith_type="Signed  (2's comp)"  n_bits=bit_width  bin_pt=bit_width-2  dbl_ovrd=off  optimize=Area  use_rpm=on  block_type=sprom
      settings: block_version=10.1.3
  sine : Outport
  cos : Outport  Port=2
  wires:
  theta/1 -> rom0/1, rom1/1
  rom0/1 -> sine/1
  rom1/1 -> cos/1

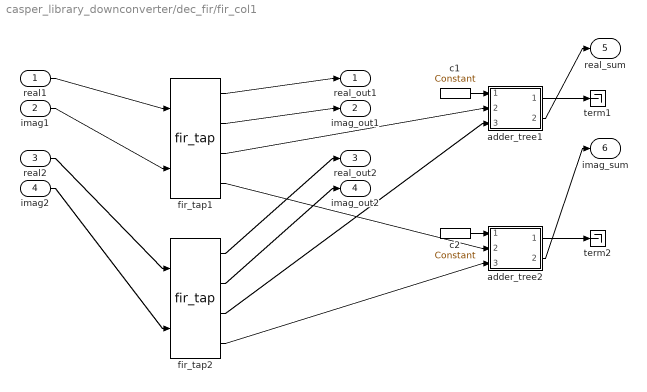
== system casper_library_downconverter/dec_fir/fir_col1 ==
  real1 : Inport
  imag1 : Inport  Port=2
  real2 : Inport  Port=3
  imag2 : Inport  Port=4
  adder_tree1 : Subsystem  AncestorBlock=casper_library_misc/adder_tree  mask(adder_tree){n_inputs=2, latency=1, first_stage_hdl=on, behavioral=off}
      mask prompts: n_inputs "Number of Inputs"; latency "Add Latency"; first_stage_hdl "Use behavioural HDL for first stage of adders"; behavioral "Use behavioral HDL for all adders"
      mask help:
      | Sums all inputs using a tree of adds and delays.
      |
      | Number of inputs: The number of inputs to the block to be summed
      | Add latency: The number of clock cycles to perform one addition (affects timing).
      | Use behavioural HDL for first stage of adders: Causes the first stage of adders to be absorbed into DSP blocks if multipliers precede them (Virtex 5).
      | Use behavioural HDL for all adders: Causes all adders in all stages to be implemented in behavioural HDL (may improve timing).
      mask init:
      | adder_tree_init(gcb, ...
      |     'n_inputs', n_inputs, ...
      |     'latency', latency, ...
      |     'first_stage_hdl', first_stage_hdl, ...
      |     'behavioral', behavioral);
      settings: AttributesFormatString=latency 1
      mask Help: eval('xlWeb(''http://casper.berkeley.edu/wiki/Adder_tree'')')
  adder_tree2 : Subsystem  AncestorBlock=casper_library_misc/adder_tree  mask(adder_tree){n_inputs=2, latency=1, first_stage_hdl=on, behavioral=off}
      mask prompts: n_inputs "Number of Inputs"; latency "Add Latency"; first_stage_hdl "Use behavioural HDL for first stage of adders"; behavioral "Use behavioral HDL for all adders"
      mask help:
      | Sums all inputs using a tree of adds and delays.
      |
      | Number of inputs: The number of inputs to the block to be summed
      | Add latency: The number of clock cycles to perform one addition (affects timing).
      | Use behavioural HDL for first stage of adders: Causes the first stage of adders to be absorbed into DSP blocks if multipliers precede them (Virtex 5).
      | Use behavioural HDL for all adders: Causes all adders in all stages to be implemented in behavioural HDL (may improve timing).
      mask init:
      | adder_tree_init(gcb, ...
      |     'n_inputs', n_inputs, ...
      |     'latency', latency, ...
      |     'first_stage_hdl', first_stage_hdl, ...
      |     'behavioral', behavioral);
      settings: AttributesFormatString=latency 1
      mask Help: eval('xlWeb(''http://casper.berkeley.edu/wiki/Adder_tree'')')
  c1 : xbsIndex_r4/Constant  arith_type=Signed (2's comp)  const=1  n_bits=16  bin_pt=14  explicit_period=on  period=1  equ=P=C  opselect=C  inp2=PCIN>>17  opr=+  inp1=P  carry=CIN  dbl_ovrd=off  block_type=constant
  c2 : xbsIndex_r4/Constant  arith_type=Signed (2's comp)  const=1  n_bits=16  bin_pt=14  explicit_period=on  period=1  equ=P=C  opselect=C  inp2=PCIN>>17  opr=+  inp1=P  carry=CIN  dbl_ovrd=off  block_type=constant
  fir_tap1 : casper_library_downconverter/fir_tap  SystemSampleTime=-1  factor=0.2  latency=2  coeff_bit_width=25  coeff_bin_pt=24
  fir_tap2 : casper_library_downconverter/fir_tap  SystemSampleTime=-1  factor=0.1  latency=2  coeff_bit_width=25  coeff_bin_pt=24
  term1 : Terminator
  term2 : Terminator
  real_out1 : Outport
  imag_out1 : Outport  Port=2
  real_out2 : Outport  Port=3
  imag_out2 : Outport  Port=4
  real_sum : Outport  Port=5
  imag_sum : Outport  Port=6
  wires:
  fir_tap2/4 -> adder_tree2/3(din2)
  fir_tap2/3 -> adder_tree1/3(din2)
  fir_tap2/2 -> imag_out2/1
  fir_tap2/1 -> real_out2/1
  imag2/1 -> fir_tap2/2
  real2/1 -> fir_tap2/1
  fir_tap1/4 -> adder_tree2/2(din1)
  fir_tap1/3 -> adder_tree1/2(din1)
  fir_tap1/2 -> imag_out1/1
  fir_tap1/1 -> real_out1/1
  imag1/1 -> fir_tap1/2
  real1/1 -> fir_tap1/1
  adder_tree2/2(dout) -> imag_sum/1
  adder_tree1/2(dout) -> real_sum/1
  c2/1 -> adder_tree2/1(sync)
  c1/1 -> adder_tree1/1(sync)
  adder_tree2/1(sync_out) -> term2/1
  adder_tree1/1(sync_out) -> term1/1

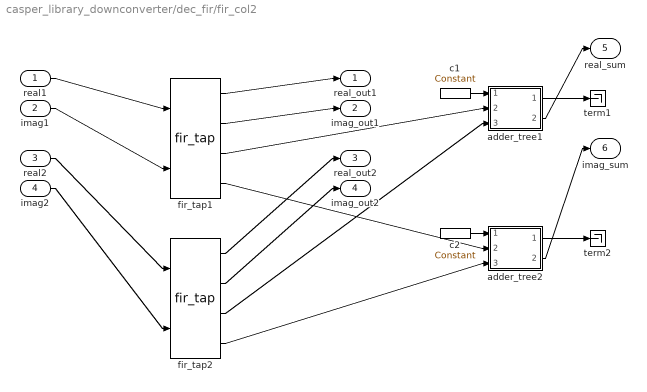
== system casper_library_downconverter/dec_fir/fir_col2 ==
  real1 : Inport
  imag1 : Inport  Port=2
  real2 : Inport  Port=3
  imag2 : Inport  Port=4
  adder_tree1 : Subsystem  AncestorBlock=casper_library_misc/adder_tree  mask(adder_tree){n_inputs=2, latency=1, first_stage_hdl=on, behavioral=off}
      mask prompts: n_inputs "Number of Inputs"; latency "Add Latency"; first_stage_hdl "Use behavioural HDL for first stage of adders"; behavioral "Use behavioral HDL for all adders"
      mask help:
      | Sums all inputs using a tree of adds and delays.
      |
      | Number of inputs: The number of inputs to the block to be summed
      | Add latency: The number of clock cycles to perform one addition (affects timing).
      | Use behavioural HDL for first stage of adders: Causes the first stage of adders to be absorbed into DSP blocks if multipliers precede them (Virtex 5).
      | Use behavioural HDL for all adders: Causes all adders in all stages to be implemented in behavioural HDL (may improve timing).
      mask init:
      | adder_tree_init(gcb, ...
      |     'n_inputs', n_inputs, ...
      |     'latency', latency, ...
      |     'first_stage_hdl', first_stage_hdl, ...
      |     'behavioral', behavioral);
      settings: AttributesFormatString=latency 1
      mask Help: eval('xlWeb(''http://casper.berkeley.edu/wiki/Adder_tree'')')
  adder_tree2 : Subsystem  AncestorBlock=casper_library_misc/adder_tree  mask(adder_tree){n_inputs=2, latency=1, first_stage_hdl=on, behavioral=off}
      mask prompts: n_inputs "Number of Inputs"; latency "Add Latency"; first_stage_hdl "Use behavioural HDL for first stage of adders"; behavioral "Use behavioral HDL for all adders"
      mask help:
      | Sums all inputs using a tree of adds and delays.
      |
      | Number of inputs: The number of inputs to the block to be summed
      | Add latency: The number of clock cycles to perform one addition (affects timing).
      | Use behavioural HDL for first stage of adders: Causes the first stage of adders to be absorbed into DSP blocks if multipliers precede them (Virtex 5).
      | Use behavioural HDL for all adders: Causes all adders in all stages to be implemented in behavioural HDL (may improve timing).
      mask init:
      | adder_tree_init(gcb, ...
      |     'n_inputs', n_inputs, ...
      |     'latency', latency, ...
      |     'first_stage_hdl', first_stage_hdl, ...
      |     'behavioral', behavioral);
      settings: AttributesFormatString=latency 1
      mask Help: eval('xlWeb(''http://casper.berkeley.edu/wiki/Adder_tree'')')
  c1 : xbsIndex_r4/Constant  arith_type=Signed (2's comp)  const=1  n_bits=16  bin_pt=14  explicit_period=on  period=1  equ=P=C  opselect=C  inp2=PCIN>>17  opr=+  inp1=P  carry=CIN  dbl_ovrd=off  block_type=constant
  c2 : xbsIndex_r4/Constant  arith_type=Signed (2's comp)  const=1  n_bits=16  bin_pt=14  explicit_period=on  period=1  equ=P=C  opselect=C  inp2=PCIN>>17  opr=+  inp1=P  carry=CIN  dbl_ovrd=off  block_type=constant
  fir_tap1 : casper_library_downconverter/fir_tap  SystemSampleTime=-1  factor=0.4  latency=2  coeff_bit_width=25  coeff_bin_pt=24
  fir_tap2 : casper_library_downconverter/fir_tap  SystemSampleTime=-1  factor=0.3  latency=2  coeff_bit_width=25  coeff_bin_pt=24
  term1 : Terminator
  term2 : Terminator
  real_out1 : Outport
  imag_out1 : Outport  Port=2
  real_out2 : Outport  Port=3
  imag_out2 : Outport  Port=4
  real_sum : Outport  Port=5
  imag_sum : Outport  Port=6
  wires:
  fir_tap2/4 -> adder_tree2/3(din2)
  fir_tap2/3 -> adder_tree1/3(din2)
  fir_tap2/2 -> imag_out2/1
  fir_tap2/1 -> real_out2/1
  imag2/1 -> fir_tap2/2
  real2/1 -> fir_tap2/1
  fir_tap1/4 -> adder_tree2/2(din1)
  fir_tap1/3 -> adder_tree1/2(din1)
  fir_tap1/2 -> imag_out1/1
  fir_tap1/1 -> real_out1/1
  imag1/1 -> fir_tap1/2
  real1/1 -> fir_tap1/1
  adder_tree2/2(dout) -> imag_sum/1
  adder_tree1/2(dout) -> real_sum/1
  c2/1 -> adder_tree2/1(sync)
  c1/1 -> adder_tree1/1(sync)
  adder_tree2/1(sync_out) -> term2/1
  adder_tree1/1(sync_out) -> term1/1

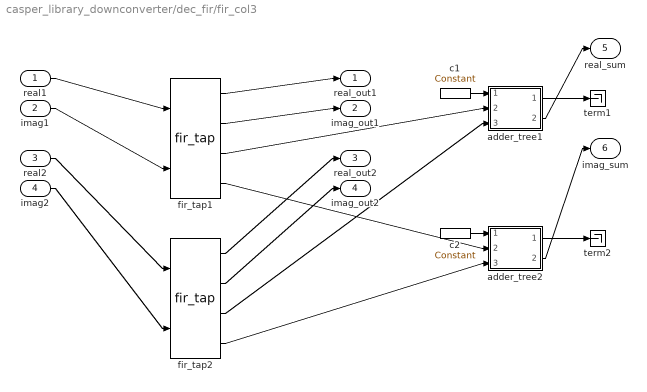
== system casper_library_downconverter/dec_fir/fir_col3 ==
  real1 : Inport
  imag1 : Inport  Port=2
  real2 : Inport  Port=3
  imag2 : Inport  Port=4
  adder_tree1 : Subsystem  AncestorBlock=casper_library_misc/adder_tree  mask(adder_tree){n_inputs=2, latency=1, first_stage_hdl=on, behavioral=off}
      mask prompts: n_inputs "Number of Inputs"; latency "Add Latency"; first_stage_hdl "Use behavioural HDL for first stage of adders"; behavioral "Use behavioral HDL for all adders"
      mask help:
      | Sums all inputs using a tree of adds and delays.
      |
      | Number of inputs: The number of inputs to the block to be summed
      | Add latency: The number of clock cycles to perform one addition (affects timing).
      | Use behavioural HDL for first stage of adders: Causes the first stage of adders to be absorbed into DSP blocks if multipliers precede them (Virtex 5).
      | Use behavioural HDL for all adders: Causes all adders in all stages to be implemented in behavioural HDL (may improve timing).
      mask init:
      | adder_tree_init(gcb, ...
      |     'n_inputs', n_inputs, ...
      |     'latency', latency, ...
      |     'first_stage_hdl', first_stage_hdl, ...
      |     'behavioral', behavioral);
      settings: AttributesFormatString=latency 1
      mask Help: eval('xlWeb(''http://casper.berkeley.edu/wiki/Adder_tree'')')
  adder_tree2 : Subsystem  AncestorBlock=casper_library_misc/adder_tree  mask(adder_tree){n_inputs=2, latency=1, first_stage_hdl=on, behavioral=off}
      mask prompts: n_inputs "Number of Inputs"; latency "Add Latency"; first_stage_hdl "Use behavioural HDL for first stage of adders"; behavioral "Use behavioral HDL for all adders"
      mask help:
      | Sums all inputs using a tree of adds and delays.
      |
      | Number of inputs: The number of inputs to the block to be summed
      | Add latency: The number of clock cycles to perform one addition (affects timing).
      | Use behavioural HDL for first stage of adders: Causes the first stage of adders to be absorbed into DSP blocks if multipliers precede them (Virtex 5).
      | Use behavioural HDL for all adders: Causes all adders in all stages to be implemented in behavioural HDL (may improve timing).
      mask init:
      | adder_tree_init(gcb, ...
      |     'n_inputs', n_inputs, ...
      |     'latency', latency, ...
      |     'first_stage_hdl', first_stage_hdl, ...
      |     'behavioral', behavioral);
      settings: AttributesFormatString=latency 1
      mask Help: eval('xlWeb(''http://casper.berkeley.edu/wiki/Adder_tree'')')
  c1 : xbsIndex_r4/Constant  arith_type=Signed (2's comp)  const=1  n_bits=16  bin_pt=14  explicit_period=on  period=1  equ=P=C  opselect=C  inp2=PCIN>>17  opr=+  inp1=P  carry=CIN  dbl_ovrd=off  block_type=constant
  c2 : xbsIndex_r4/Constant  arith_type=Signed (2's comp)  const=1  n_bits=16  bin_pt=14  explicit_period=on  period=1  equ=P=C  opselect=C  inp2=PCIN>>17  opr=+  inp1=P  carry=CIN  dbl_ovrd=off  block_type=constant
  fir_tap1 : casper_library_downconverter/fir_tap  SystemSampleTime=-1  factor=0.6  latency=2  coeff_bit_width=25  coeff_bin_pt=24
  fir_tap2 : casper_library_downconverter/fir_tap  SystemSampleTime=-1  factor=0.5  latency=2  coeff_bit_width=25  coeff_bin_pt=24
  term1 : Terminator
  term2 : Terminator
  real_out1 : Outport
  imag_out1 : Outport  Port=2
  real_out2 : Outport  Port=3
  imag_out2 : Outport  Port=4
  real_sum : Outport  Port=5
  imag_sum : Outport  Port=6
  wires:
  fir_tap2/4 -> adder_tree2/3(din2)
  fir_tap2/3 -> adder_tree1/3(din2)
  fir_tap2/2 -> imag_out2/1
  fir_tap2/1 -> real_out2/1
  imag2/1 -> fir_tap2/2
  real2/1 -> fir_tap2/1
  fir_tap1/4 -> adder_tree2/2(din1)
  fir_tap1/3 -> adder_tree1/2(din1)
  fir_tap1/2 -> imag_out1/1
  fir_tap1/1 -> real_out1/1
  imag1/1 -> fir_tap1/2
  real1/1 -> fir_tap1/1
  adder_tree2/2(dout) -> imag_sum/1
  adder_tree1/2(dout) -> real_sum/1
  c2/1 -> adder_tree2/1(sync)
  c1/1 -> adder_tree1/1(sync)
  adder_tree2/1(sync_out) -> term2/1
  adder_tree1/1(sync_out) -> term1/1
